simulink model "model_axe3_BF"  (Simulink 8.3)
settings: Solver=ode5  StartTime=0.0  StopTime=tsim  FixedStep=Fixed_Step  MaxStep=time_step  RelTol=1e-3
values from neighbouring files (symbols this model uses):
  Choix = 5    [Traces_BF.m]    (also in traces.m)
  Cs1n = 0    [data_gyros.m]
  Cs2n = 0    [data_gyros.m]
  Cs3n = 0    [data_gyros.m]
  Cs4n = 0    [data_gyros.m]
  Fixed_Step = 0.01    [Traces_BF.m]    (also in traces.m)
  K1 = 6667/(2*pi)    (= 1061.08600559)    [data_gyros.m]    (also in gyro_data.m)
  K2 = 24400/(2*pi)    (= 3883.38061144)    [data_gyros.m]    (also in gyro_data.m)
  K3 = 16000/(2*pi)    (= 2546.47908947)    [data_gyros.m]    (also in gyro_data.m)
  K4 = 16000/(2*pi)    (= 2546.47908947)    [data_gyros.m]    (also in gyro_data.m)
  Kamp = 0.4    [data_gyros.m]    (also in gyro_data.m)
  Kg = 1/2*wn/zeta    (= 21.4285714286)    [Traces_BF.m]    (also in traces.m)
  Km1 = 0.175    [data_gyros.m]    (also in gyro_data.m)
  Km2 = 0.732    [data_gyros.m]    (also in gyro_data.m)
  Kpv = 2*(Ic+Id)*wn*zeta    [Traces_BF.m]    (also in traces.m)
  mu1n = 0    [data_gyros.m]
  mu1p = 0    [data_gyros.m]
  mu2n = 0    [data_gyros.m]
  mu2p = 0    [data_gyros.m]
  mu3n = 0    [data_gyros.m]
  mu3p = 0    [data_gyros.m]
  mu4n = 0    [data_gyros.m]
  mu4p = 0    [data_gyros.m]
  Omega1_0 = 0    [Traces_BF.m]    (also in data_gyros.m; traces.m)
  Omega1_c = 500    [Traces_BF.m]    (also in traces.m)
  Omega2_0 = 0    [Traces_BF.m]    (also in data_gyros.m; traces.m)
  q20 = pi/2    (= 1.57079632679)    [Traces_BF.m]    (also in traces.m)
  q30 = 0    [Traces_BF.m]    (also in traces.m)
  Theta2_c = 0    [Traces_BF.m]    (also in traces.m)
undefined symbols (not defined in the file or in its folder): A, B, C, consigne_sin_q3, D, frequence_sin_q3, Kd, Kp, Kv1, Theta3_c
libraries: simulink x8, library_gyro x1
settings Model: Creator=CrazySix  LastModifiedBy=ahmed.chaibet
settings DataIOCC: LimitDataPoints=off
settings OptimizationCC: BooleanDataType=off  ExpressionDepthLimit=2147483647
settings DebuggingCC: SaveWithParameterizedLinksMsg=none  SignalResolutionControl=TryResolveAllWithWarning  SolverPrmCheckMsg=none  MultiTaskDSMMsg=warning  MultiTaskCondExecSysMsg=none  FcnCallInpInsideContextMsg=UseLocalSettings  StrictBusMsg=None
settings HardwareCC: TargetUnknown=on
settings RTWCC: IncludeERTFirstTime=on

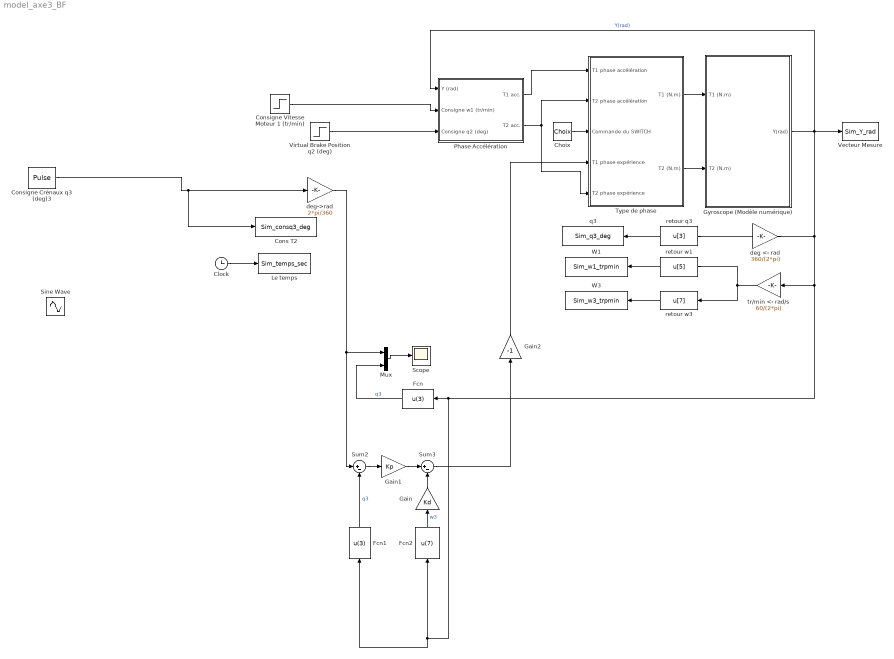
== system model_axe3_BF ==
  Choix : Constant  Value=Choix
  Clock : Clock
  Cons T2 : ToWorkspace  VariableName=Sim_consq3_deg  SampleTime=-1
  Consigne Crénaux q3 (deg)3 : DiscretePulseGenerator  PulseType=Time based  Amplitude=Theta3_c  Period=10  PulseWidth=50  SampleTime=Fixed_Step
  Consigne Vitesse Moteur 1 (tr/min) : Step  Time=0  Before=Omega1_c  After=0  SampleTime=0
  Fcn : Fcn  Expr=u(3)
  Fcn1 : Fcn  Expr=u(3)
  Fcn2 : Fcn  Expr=u(7)
  Gain : Gain  Gain=Kd  SaturateOnIntegerOverflow=on  OutDataTypeStr=Inherit: Same as input  ParamDataTypeStr=Inherit: Same as input
  Gain1 : Gain  Gain=Kp  SaturateOnIntegerOverflow=on  OutDataTypeStr=Inherit: Same as input  ParamDataTypeStr=Inherit: Same as input
  Gain2 : Gain  Gain=-1  SaturateOnIntegerOverflow=on  OutDataTypeStr=Inherit: Same as input  ParamDataTypeStr=Inherit: Same as input
  Gyroscope (Modèle numérique) : Subsystem
  Le temps : ToWorkspace  VariableName=Sim_temps_sec  SampleTime=-1
  Mux : Mux  Inputs=2
  Phase Accélération : Subsystem
  Scope : Scope
      settings: YMin=0  YMax=0.09
  Sine Wave : Sin  Amplitude=consigne_sin_q3  Frequency=frequence_sin_q3  SampleTime=0
  Sum2 : Sum  Inputs=|+-  SaturateOnIntegerOverflow=on  InputSameDT=on  OutDataTypeStr=Inherit: Same as first input
  Sum3 : Sum  Inputs=|+-  SaturateOnIntegerOverflow=on  InputSameDT=on  OutDataTypeStr=Inherit: Same as first input
  Type de phase : Subsystem
  Vecteur Mesure : ToWorkspace  VariableName=Sim_Y_rad  SampleTime=-1
  Virtual Brake Position q2 (deg) : Step  Time=0  Before=Theta2_c  After=0  SampleTime=0
  W1 : ToWorkspace  VariableName=Sim_w1_trpmin  SampleTime=-1
  W3 : ToWorkspace  VariableName=Sim_w3_trpmin  SampleTime=-1
  deg <- rad : Gain  Gain=360/(2*pi)  SaturateOnIntegerOverflow=on  OutDataTypeStr=Inherit: Same as input  ParamDataTypeStr=Inherit: Same as input
  deg->rad : Gain  Gain=2*pi/360  SaturateOnIntegerOverflow=on  OutDataTypeStr=Inherit: Same as input  ParamDataTypeStr=Inherit: Same as input
  q3 : ToWorkspace  VariableName=Sim_q3_deg  SampleTime=-1
  retour q3 : Fcn  Expr=u[3]
  retour w1 : Fcn  Expr=u[5]
  retour w3 : Fcn  Expr=u[7]
  tr/min <- rad/s : Gain  Gain=60/(2*pi)  SaturateOnIntegerOverflow=on  OutDataTypeStr=Inherit: Same as input  ParamDataTypeStr=Inherit: Same as input
  wires:
  Clock/1 -> Le temps/1
  Gyroscope (Modèle numérique)/1(Y(rad)) -> Vecteur Mesure/1, deg <- rad/1, tr/min <- rad/s/1, Fcn2/1, Fcn1/1, Fcn/1, Phase Accélération/1(Y (rad))  "Y(rad)"
  tr/min <- rad/s/1 -> retour w1/1, retour w3/1
  retour w1/1 -> W1/1
  retour w3/1 -> W3/1
  Consigne Vitesse Moteur 1 (tr/min)/1 -> Phase Accélération/2("Consigne w1 (tr/min) ")
  Virtual Brake Position q2 (deg)/1 -> Phase Accélération/3("Consigne q2 (deg) ")
  Phase Accélération/2(T2 acc.) -> Type de phase/2(T2 phase accélération), Type de phase/5(T2 phase expérience)
  Phase Accélération/1(T1 acc.) -> Type de phase/1(T1 phase accélération)
  Choix/1 -> Type de phase/3(Commande du SWITCH)
  Type de phase/1(T1 (N.m)) -> Gyroscope (Modèle numérique)/1(T1 (N.m))
  Type de phase/2(T2 (N.m)) -> Gyroscope (Modèle numérique)/2(T2 (N.m))
  retour q3/1 -> q3/1
  deg <- rad/1 -> retour q3/1
  Mux/1 -> Scope/1
  Fcn/1 -> Mux/2  "q3"
  Sum2/1 -> Gain1/1
  Fcn1/1 -> Sum2/2  "q3"
  Gain/1 -> Sum3/2
  Fcn2/1 -> Gain/1  "w3"
  deg->rad/1 -> Mux/1, Sum2/1
  Gain1/1 -> Sum3/1
  Sum3/1 -> Gain2/1
  Gain2/1 -> Type de phase/4(T1 phase expérience)
  Consigne Crénaux q3 (deg)3/1 -> Cons T2/1, deg->rad/1

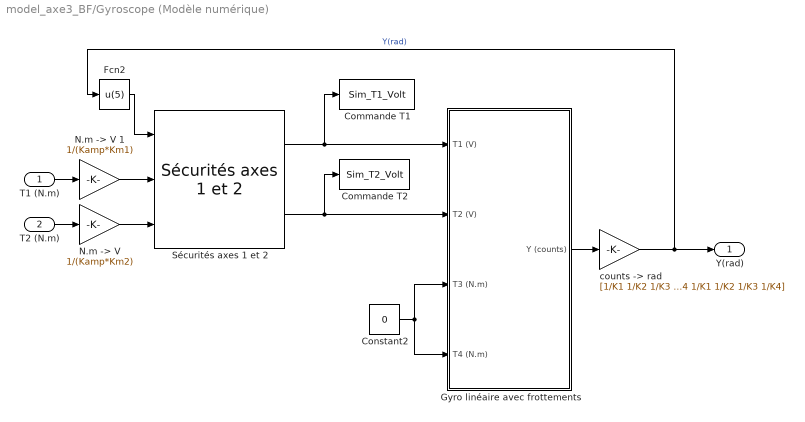
== system model_axe3_BF/Gyroscope (Modèle numérique) ==
  T1 (N.m) : Inport
  T2 (N.m) : Inport  Port=2
  Commande T1 : ToWorkspace  VariableName=Sim_T1_Volt  SampleTime=-1
  Commande T2 : ToWorkspace  VariableName=Sim_T2_Volt  SampleTime=-1
  Constant2 : Constant  Value=0
  Fcn2 : Fcn  Expr=u(5)
  Gyro linéaire avec frottements : Subsystem
  "N.m -> V" : Gain  Gain=1/(Kamp*Km2)  SaturateOnIntegerOverflow=on  OutDataTypeStr=Inherit: Same as input  ParamDataTypeStr=Inherit: Same as input
  "N.m -> V 1" : Gain  Gain=1/(Kamp*Km1)  SaturateOnIntegerOverflow=on  OutDataTypeStr=Inherit: Same as input  ParamDataTypeStr=Inherit: Same as input
  Sécurités axes 1 et 2 : library_gyro/Sécurités axes 1 et 2
  "counts -> rad" : Gain  Gain=[1/K1 1/K2 1/K3 1/K4 1/K1 1/K2 1/K3 1/K4]  SaturateOnIntegerOverflow=on  OutDataTypeStr=Inherit: Same as input  ParamDataTypeStr=Inherit: Same as input
  Y(rad) : Outport
  wires:
  Gyro linéaire avec frottements/1(Y (counts)) -> "counts -> rad"/1
  Sécurités axes 1 et 2/2 -> Gyro linéaire avec frottements/2(T2 (V)), Commande T2/1
  Sécurités axes 1 et 2/1 -> Gyro linéaire avec frottements/1(T1 (V)), Commande T1/1
  Constant2/1 -> Gyro linéaire avec frottements/4(T4 (N.m)), Gyro linéaire avec frottements/3(T3 (N.m))
  "N.m -> V"/1 -> Sécurités axes 1 et 2/3
  "counts -> rad"/1 -> Y(rad)/1, Fcn2/1  "Y(rad)"
  Fcn2/1 -> Sécurités axes 1 et 2/1
  "N.m -> V 1"/1 -> Sécurités axes 1 et 2/2
  T1 (N.m)/1 -> "N.m -> V 1"/1
  T2 (N.m)/1 -> "N.m -> V"/1

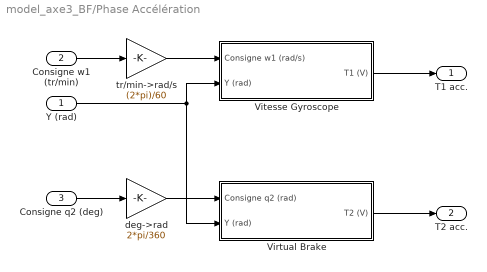
== system model_axe3_BF/Phase Accélération ==
  Y (rad) : Inport
  "Consigne w1 (tr/min) " : Inport  Port=2
  "Consigne q2 (deg) " : Inport  Port=3
  Virtual Brake : Subsystem
  Vitesse Gyroscope : Subsystem
  deg->rad : Gain  Gain=2*pi/360  SaturateOnIntegerOverflow=on  OutDataTypeStr=Inherit: Same as input  ParamDataTypeStr=Inherit: Same as input
  tr/min->rad/s : Gain  Gain=(2*pi)/60  SaturateOnIntegerOverflow=on  OutDataTypeStr=Inherit: Same as input  ParamDataTypeStr=Inherit: Same as input
  T1 acc. : Outport
  T2 acc. : Outport  Port=2
  wires:
  Y (rad)/1 -> Virtual Brake/2(Y (rad)), Vitesse Gyroscope/2(Y (rad))
  "Consigne q2 (deg) "/1 -> deg->rad/1
  Vitesse Gyroscope/1(T1 (V)) -> T1 acc./1
  Virtual Brake/1(T2 (V)) -> T2 acc./1
  tr/min->rad/s/1 -> Vitesse Gyroscope/1("Consigne w1 (rad/s) ")
  "Consigne w1 (tr/min) "/1 -> tr/min->rad/s/1
  deg->rad/1 -> Virtual Brake/1("Consigne q2 (rad) ")

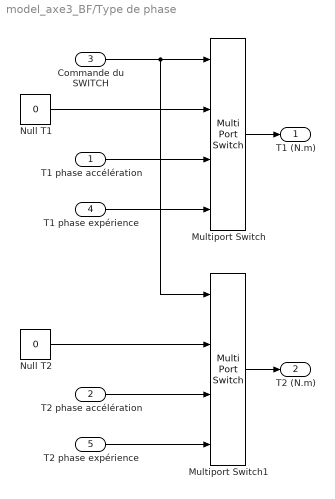
== system model_axe3_BF/Type de phase ==
  T1 phase accélération : Inport
  T2 phase accélération : Inport  Port=2
  Commande du SWITCH : Inport  Port=3
  T1 phase expérience : Inport  Port=4
  T2 phase expérience : Inport  Port=5
  Multiport Switch : MultiPortSwitch  SaturateOnIntegerOverflow=on  InputSameDT=on
  Multiport Switch1 : MultiPortSwitch  SaturateOnIntegerOverflow=on  InputSameDT=on
  Null T1 : Constant  Value=0
  Null T2 : Constant  Value=0
  T1 (N.m) : Outport
  T2 (N.m) : Outport  Port=2
  wires:
  Multiport Switch/1 -> T1 (N.m)/1
  Commande du SWITCH/1 -> Multiport Switch/1, Multiport Switch1/1
  Multiport Switch1/1 -> T2 (N.m)/1
  T2 phase expérience/1 -> Multiport Switch1/4
  T2 phase accélération/1 -> Multiport Switch1/3
  T1 phase expérience/1 -> Multiport Switch/4
  T1 phase accélération/1 -> Multiport Switch/3
  Null T1/1 -> Multiport Switch/2
  Null T2/1 -> Multiport Switch1/2

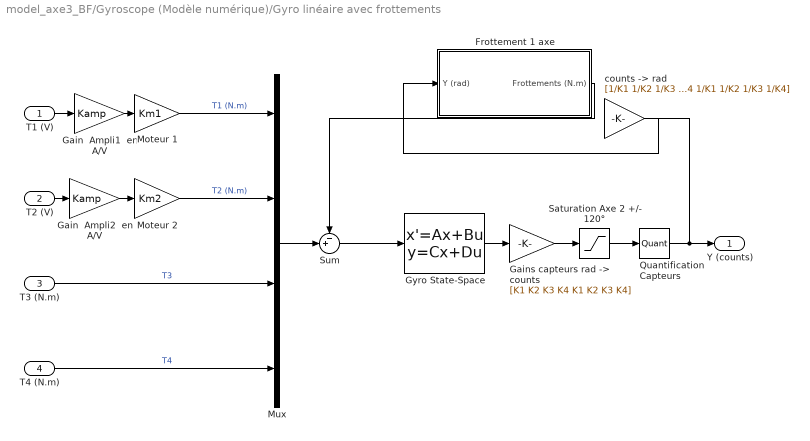
== system model_axe3_BF/Gyroscope (Modèle numérique)/Gyro linéaire avec frottements ==
  T1 (V) : Inport
  T2 (V) : Inport  Port=2
  T3 (N.m) : Inport  Port=3
  T4 (N.m) : Inport  Port=4
  Frottement 1 axe : Subsystem
  Gain  Ampli1  en A/V : Gain  Gain=Kamp  SaturateOnIntegerOverflow=on  OutDataTypeStr=Inherit: Same as input  ParamDataTypeStr=Inherit: Same as input
  Gain  Ampli2  en A/V : Gain  Gain=Kamp  SaturateOnIntegerOverflow=on  OutDataTypeStr=Inherit: Same as input  ParamDataTypeStr=Inherit: Same as input
  "Gains capteurs rad -> counts" : Gain  Gain=[K1 K2 K3 K4 K1 K2 K3 K4]  SaturateOnIntegerOverflow=on  OutDataTypeStr=Inherit: Same as input  ParamDataTypeStr=Inherit: Same as input
  Gyro State-Space : StateSpace  A=A  B=B  C=C  D=D  X0=[0 q20 q30 0 Omega1_0 Omega2_0 0 0]
  Moteur 1 : Gain  Gain=Km1  SaturateOnIntegerOverflow=on  OutDataTypeStr=Inherit: Same as input  ParamDataTypeStr=Inherit: Same as input
  Moteur 2 : Gain  Gain=Km2  SaturateOnIntegerOverflow=on  OutDataTypeStr=Inherit: Same as input  ParamDataTypeStr=Inherit: Same as input
  Mux : Mux
  Quantification Capteurs : Quantizer  QuantizationInterval=Q
  Saturation Axe 2 +/- 120° : Saturate  UpperLimit=[inf 120*pi/180*K2 inf inf inf inf inf inf]  LowerLimit=[-inf -120*pi/180*K2 -inf -inf -inf -inf -inf -inf]
  Sum : Sum  Inputs=-+|  SaturateOnIntegerOverflow=on  InputSameDT=on  OutDataTypeStr=Inherit: Same as first input
  "counts -> rad" : Gain  Gain=[1/K1 1/K2 1/K3 1/K4 1/K1 1/K2 1/K3 1/K4]  SaturateOnIntegerOverflow=on  OutDataTypeStr=Inherit: Same as input  ParamDataTypeStr=Inherit: Same as input
  Y (counts) : Outport
  wires:
  T1 (V)/1 -> Gain  Ampli1  en A/V/1
  Gain  Ampli1  en A/V/1 -> Moteur 1/1
  Moteur 2/1 -> Mux/2  "T2 (N.m)"
  Gain  Ampli2  en A/V/1 -> Moteur 2/1
  Gyro State-Space/1 -> "Gains capteurs rad -> counts"/1
  T2 (V)/1 -> Gain  Ampli2  en A/V/1
  Saturation Axe 2 +/- 120°/1 -> Quantification Capteurs/1
  Quantification Capteurs/1 -> Y (counts)/1, "counts -> rad"/1
  T3 (N.m)/1 -> Mux/3  "T3"
  T4 (N.m)/1 -> Mux/4  "T4"
  "Gains capteurs rad -> counts"/1 -> Saturation Axe 2 +/- 120°/1
  Moteur 1/1 -> Mux/1  "T1 (N.m)"
  Mux/1 -> Sum/2
  Sum/1 -> Gyro State-Space/1
  Frottement 1 axe/1(Frottements (N.m)) -> Sum/1
  "counts -> rad"/1 -> Frottement 1 axe/1(Y (rad))

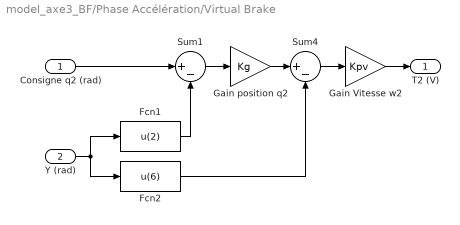
== system model_axe3_BF/Phase Accélération/Virtual Brake ==
  "Consigne q2 (rad) " : Inport
  Y (rad) : Inport  Port=2
  Fcn1 : Fcn  Expr=u(2)
  Fcn2 : Fcn  Expr=u(6)
  Gain Vitesse w2 : Gain  Gain=Kpv  SaturateOnIntegerOverflow=on  OutDataTypeStr=Inherit: Same as input  ParamDataTypeStr=Inherit: Same as input
  Gain position q2 : Gain  Gain=Kg  SaturateOnIntegerOverflow=on  OutDataTypeStr=Inherit: Same as input  ParamDataTypeStr=Inherit: Same as input
  Sum1 : Sum  Inputs=|+-  SaturateOnIntegerOverflow=on  InputSameDT=on  OutDataTypeStr=Inherit: Same as first input
  Sum4 : Sum  Inputs=|+-  SaturateOnIntegerOverflow=on  InputSameDT=on  OutDataTypeStr=Inherit: Same as first input
  T2 (V) : Outport
  wires:
  Fcn1/1 -> Sum1/2
  Sum1/1 -> Gain position q2/1
  Sum4/1 -> Gain Vitesse w2/1
  Fcn2/1 -> Sum4/2
  "Consigne q2 (rad) "/1 -> Sum1/1
  Gain position q2/1 -> Sum4/1
  Y (rad)/1 -> Fcn2/1, Fcn1/1
  Gain Vitesse w2/1 -> T2 (V)/1

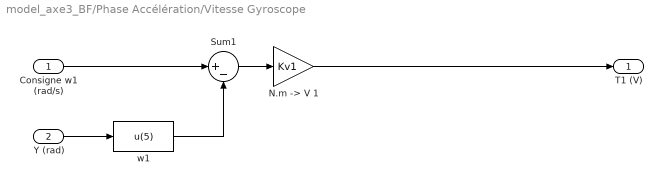
== system model_axe3_BF/Phase Accélération/Vitesse Gyroscope ==
  "Consigne w1 (rad/s) " : Inport
  Y (rad) : Inport  Port=2
  "N.m -> V 1" : Gain  Gain=Kv1  SaturateOnIntegerOverflow=on  OutDataTypeStr=Inherit: Same as input  ParamDataTypeStr=Inherit: Same as input
  Sum1 : Sum  Inputs=|+-  SaturateOnIntegerOverflow=on  InputSameDT=on  OutDataTypeStr=Inherit: Same as first input
  w1 : Fcn  Expr=u(5)
  T1 (V) : Outport
  wires:
  w1/1 -> Sum1/2
  Sum1/1 -> "N.m -> V 1"/1
  "Consigne w1 (rad/s) "/1 -> Sum1/1
  Y (rad)/1 -> w1/1
  "N.m -> V 1"/1 -> T1 (V)/1

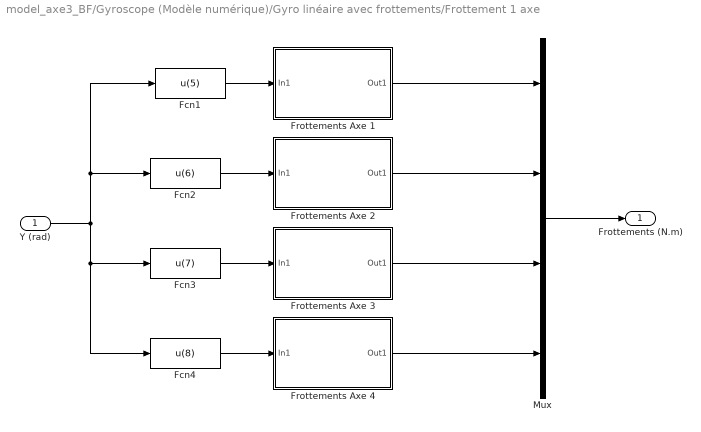
== system model_axe3_BF/Gyroscope (Modèle numérique)/Gyro linéaire avec frottements/Frottement 1 axe ==
  Y (rad) : Inport
  Fcn1 : Fcn  Expr=u(5)
  Fcn2 : Fcn  Expr=u(6)
  Fcn3 : Fcn  Expr=u(7)
  Fcn4 : Fcn  Expr=u(8)
  Frottements Axe 1 : Subsystem
  Frottements Axe 2 : Subsystem
  Frottements Axe 3 : Subsystem
  Frottements Axe 4 : Subsystem
  Mux : Mux
  Frottements (N.m) : Outport
  wires:
  Frottements Axe 1/1(Out1) -> Mux/1
  Y (rad)/1 -> Fcn1/1, Fcn2/1, Fcn3/1, Fcn4/1
  Fcn1/1 -> Frottements Axe 1/1(In1)
  Fcn4/1 -> Frottements Axe 4/1(In1)
  Fcn3/1 -> Frottements Axe 3/1(In1)
  Mux/1 -> Frottements (N.m)/1
  Frottements Axe 3/1(Out1) -> Mux/3
  Frottements Axe 4/1(Out1) -> Mux/4
  Fcn2/1 -> Frottements Axe 2/1(In1)
  Frottements Axe 2/1(Out1) -> Mux/2

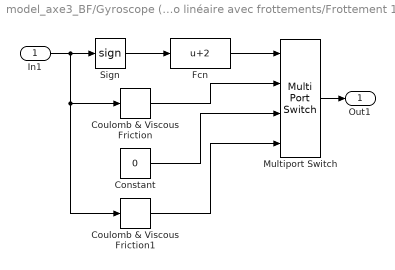
== system model_axe3_BF/Gyroscope (Modèle numérique)/Gyro linéaire avec frottements/Frottement 1 axe/Frottements Axe 1 ==
  In1 : Inport
  Constant : Constant  Value=0
  Coulomb & Viscous Friction : simulink/Discontinuities/Coulomb & Viscous Friction  offset=abs(Cs1n)  gain=mu1n
  Coulomb & Viscous Friction1 : simulink/Discontinuities/Coulomb & Viscous Friction  offset=Cs1p  gain=mu1p
  Fcn : Fcn  Expr=u+2
  Multiport Switch : MultiPortSwitch  SaturateOnIntegerOverflow=on  InputSameDT=on
  Sign : Signum
  Out1 : Outport
  wires:
  In1/1 -> Sign/1, Coulomb & Viscous Friction/1, Coulomb & Viscous Friction1/1
  Fcn/1 -> Multiport Switch/1
  Sign/1 -> Fcn/1
  Coulomb & Viscous Friction1/1 -> Multiport Switch/4
  Constant/1 -> Multiport Switch/3
  Coulomb & Viscous Friction/1 -> Multiport Switch/2
  Multiport Switch/1 -> Out1/1

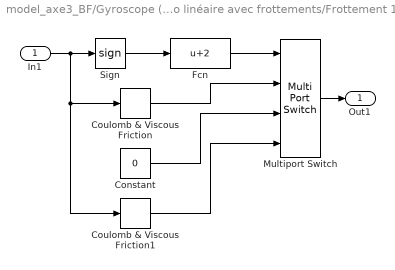
== system model_axe3_BF/Gyroscope (Modèle numérique)/Gyro linéaire avec frottements/Frottement 1 axe/Frottements Axe 2 ==
  In1 : Inport
  Constant : Constant  Value=0
  Coulomb & Viscous Friction : simulink/Discontinuities/Coulomb & Viscous Friction  offset=abs(Cs2n)  gain=mu2n
  Coulomb & Viscous Friction1 : simulink/Discontinuities/Coulomb & Viscous Friction  offset=Cs2p  gain=mu2p
  Fcn : Fcn  Expr=u+2
  Multiport Switch : MultiPortSwitch  SaturateOnIntegerOverflow=on  InputSameDT=on
  Sign : Signum
  Out1 : Outport
  wires:
  Multiport Switch/1 -> Out1/1
  Coulomb & Viscous Friction/1 -> Multiport Switch/2
  Constant/1 -> Multiport Switch/3
  Coulomb & Viscous Friction1/1 -> Multiport Switch/4
  Sign/1 -> Fcn/1
  Fcn/1 -> Multiport Switch/1
  In1/1 -> Coulomb & Viscous Friction1/1, Coulomb & Viscous Friction/1, Sign/1

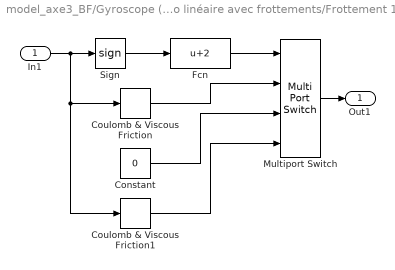
== system model_axe3_BF/Gyroscope (Modèle numérique)/Gyro linéaire avec frottements/Frottement 1 axe/Frottements Axe 3 ==
  In1 : Inport
  Constant : Constant  Value=0
  Coulomb & Viscous Friction : simulink/Discontinuities/Coulomb & Viscous Friction  offset=abs(Cs3n)  gain=mu3n
  Coulomb & Viscous Friction1 : simulink/Discontinuities/Coulomb & Viscous Friction  offset=Cs3p  gain=mu3p
  Fcn : Fcn  Expr=u+2
  Multiport Switch : MultiPortSwitch  SaturateOnIntegerOverflow=on  InputSameDT=on
  Sign : Signum
  Out1 : Outport
  wires:
  In1/1 -> Sign/1, Coulomb & Viscous Friction/1, Coulomb & Viscous Friction1/1
  Fcn/1 -> Multiport Switch/1
  Sign/1 -> Fcn/1
  Coulomb & Viscous Friction1/1 -> Multiport Switch/4
  Constant/1 -> Multiport Switch/3
  Coulomb & Viscous Friction/1 -> Multiport Switch/2
  Multiport Switch/1 -> Out1/1

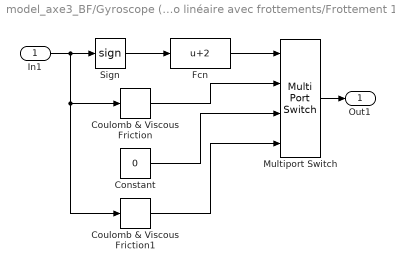
== system model_axe3_BF/Gyroscope (Modèle numérique)/Gyro linéaire avec frottements/Frottement 1 axe/Frottements Axe 4 ==
  In1 : Inport
  Constant : Constant  Value=0
  Coulomb & Viscous Friction : simulink/Discontinuities/Coulomb & Viscous Friction  offset=abs(Cs4n)  gain=mu4n
  Coulomb & Viscous Friction1 : simulink/Discontinuities/Coulomb & Viscous Friction  offset=Cs4p  gain=mu4p
  Fcn : Fcn  Expr=u+2
  Multiport Switch : MultiPortSwitch  SaturateOnIntegerOverflow=on  InputSameDT=on
  Sign : Signum
  Out1 : Outport
  wires:
  Multiport Switch/1 -> Out1/1
  Coulomb & Viscous Friction/1 -> Multiport Switch/2
  Constant/1 -> Multiport Switch/3
  Coulomb & Viscous Friction1/1 -> Multiport Switch/4
  Sign/1 -> Fcn/1
  Fcn/1 -> Multiport Switch/1
  In1/1 -> Coulomb & Viscous Friction1/1, Coulomb & Viscous Friction/1, Sign/1
